simulink library "UsefulBlocksLibrary"  (R2014b)
settings: Solver=ode45  SolverMode=SingleTasking  StartTime=0.0  StopTime=10.0  RelTol=1e-3
undefined symbols (not defined in the file): ActuatorStruct, CalibrationAngles, drivePeakCurrent, JointAbsoluteEncoderCounts_rev, JointPositionGuardMax_rad, JointPositionGuardMin_rad, MotorEncoderCounts_rev, motorTorqueConstant, sampleTime, transmissionRatio
libraries: simulink x13, FM_Library x4, dspsigops x1, simulink_extras x1
(part 1 of 2)
settings Model: Creator=niekbeckers  LastModifiedBy=Administrator
settings OptimizationCC: BlockReduction=off  BooleanDataType=off  UseDivisionForNetSlopeComputation=off  SimCompilerOptimization=off
settings DebuggingCC: SaveWithParameterizedLinksMsg=none  UnderspecifiedInitializationDetection=Classic  MergeDetectMultiDrivingBlocksExec=none  SignalResolutionControl=TryResolveAllWithWarning  SolverPrmCheckMsg=none  FrameProcessingCompatibilityMsg=error  StrictBusMsg=Warning
settings HardwareCC: TargetUnknown=on
settings RTWCC: RTWCompilerOptimization=off
settings ConfigComp: CovMetricSettings=dw  CovHtmlReporting=on  CovSaveCumulativeToWorkspaceVar=on  CovSaveSingleToWorkspaceVar=on  CovModelRefEnable=Off  CovExternalEMLEnable=off  CovSFcnEnable=off

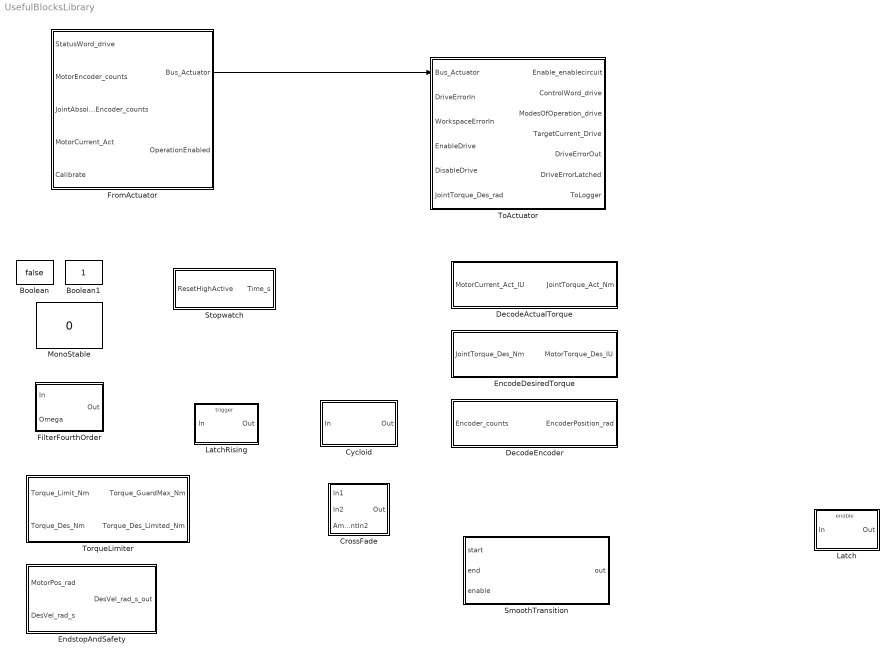
== system UsefulBlocksLibrary ==
  Boolean : Constant  Value=false  OutDataTypeStr=boolean
      settings: OpenFcn=|
      | b = get_param(gcb,'value');
      | if (strcmp(b,'true')),
      |   set_param (gcb,'value','false');
      | else
      |   set_param(gcb,'value','true');
      | end;
  Boolean1 : Constant  OutDataTypeStr=double
      settings: OpenFcn=|
      | b = get_param(gcb,'value');
      | if (strcmp(b,'1')),
      |   set_param (gcb,'value','0');
      | else
      |   set_param(gcb,'value','1');
      | end;
  CrossFade : Subsystem
  Cycloid : Subsystem
  DecodeActualTorque : MATLAB Function  TreatAsAtomicUnit=on  mask(DecodeActualTorque){transmissionRatio=transmissionRatio, motorTorqueConstant=motorTorqueConstant, drivePeakCurrent=drivePeakCurrent}
      mask prompts: transmissionRatio "Transmission ratio (e.g. -8) [-]"; motorTorqueConstant "Motor torque constant [Nm/A]"; drivePeakCurrent "Motor drive peak current Ipeak [A]"
      mask help:
      | Decode Actual Torque value returned from the actuator (motor drive and motor) to torque on the joint (after transmission).
      |
      | Note: due to the way the transmission is set up and the positive motor axis (clockwise is positive as seen from the motor front), there is no need to account for sign change in motor torque or encoder position.
  DecodeEncoder : MATLAB Function  TreatAsAtomicUnit=on  mask(DecodeEncoder){EncoderCounts_rev=MotorEncoderCounts_rev}
      mask prompts: EncoderCounts_rev "Motor encoder increments per revolution (e.g., 8192)"
      mask help: Decode the encoder counts to encoder position in radians
  EncodeDesiredTorque : MATLAB Function  TreatAsAtomicUnit=on  mask(EncodeDesiredTorque){transmissionRatio=transmissionRatio, motorTorqueConstant=motorTorqueConstant, drivePeakCurrent=drivePeakCurrent}
      mask prompts: transmissionRatio "Transmission ratio (e.g. -8) [-]"; motorTorqueConstant "Motor torque constant [Nm/A]"; drivePeakCurrent "Motor drive peak current [A]"
      mask help:
      | Encode desired torque at the joint to torque to be produced by the motor.
      |
      | Note: due to the way the transmission is set up and the positive motor axis (clockwise is positive as seen from the motor front), there is no need to account for sign change in motor torque or encoder position.
  EndstopAndSafety : Subsystem
  FilterFourthOrder : Subsystem
  FromActuator : Subsystem  mask{IdxJoint=1}
      mask prompts: IdxJoint "Actuator joint number (1 = q1, 2 = q5)"
  Latch : Subsystem  mask{ic=0}
      mask prompts: ic "Initial Condition"
  LatchRising : Subsystem  mask{ic=0}
      mask prompts: ic "Initial Condition"
  MonoStable : Constant  Value=0
      settings: OpenFcn=set_param(gcb,'Value','1');tname = ['toggletimer_' gcb];delete(timerfind('name',tname));t = timer('timerfcn', ['set_param(''',gcb,''',''Value'',''0'')'],'executionmode','singleshot','startdelay',1,'name',tname);start(t);
      mask Display: fprintf('PushToTrigger\n%s',get_param(gcb,'value'))
  SmoothTransition : Subsystem
  Stopwatch : Subsystem
  ToActuator : Subsystem  mask{IdxJoint=1}
      mask prompts: IdxJoint "Actuator joint number (1 = q1, 2 = q5)"
  TorqueLimiter : Subsystem
  wires:
  FromActuator/1(Bus_Actuator) -> ToActuator/1(Bus_Actuator)

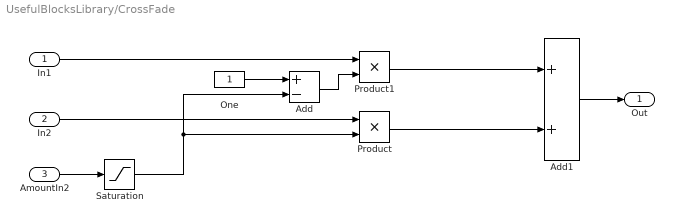
== system UsefulBlocksLibrary/CrossFade ==
  In1 : Inport
  In2 : Inport  Port=2
  AmountIn2 : Inport  Port=3
  Add : Sum  Inputs=+-
  Add1 : Sum
  One : Constant
  Product : Product  RndMeth=Zero
  Product1 : Product  RndMeth=Zero
  Saturation : Saturate  UpperLimit=1  LowerLimit=0
  Out : Outport
  wires:
  In1/1 -> Product1/1
  AmountIn2/1 -> Saturation/1
  One/1 -> Add/1
  Saturation/1 -> Product/2, Add/2
  Add/1 -> Product1/2
  Product/1 -> Add1/2
  Product1/1 -> Add1/1
  In2/1 -> Product/1
  Add1/1 -> Out/1

== system UsefulBlocksLibrary/Cycloid ==
  note: Given a linear input 0<=in<=1, it gives a cycloid output 0<=out<=1.
      | If In is outside the 0..1 range, it is limited to 0 or 1.
  In : Inport
  Gain1 : Gain  Gain=2*pi
  Gain2 : Gain  Gain=1/(2*pi)
  Saturation : Saturate  UpperLimit=1  LowerLimit=0
  Subtract : Sum  Inputs=+-
  Trigonometric Function : Trigonometry
  Out : Outport
  wires:
  Gain1/1 -> Trigonometric Function/1
  Subtract/1 -> Out/1
  In/1 -> Saturation/1
  Saturation/1 -> Gain1/1, Subtract/1
  Trigonometric Function/1 -> Gain2/1
  Gain2/1 -> Subtract/2

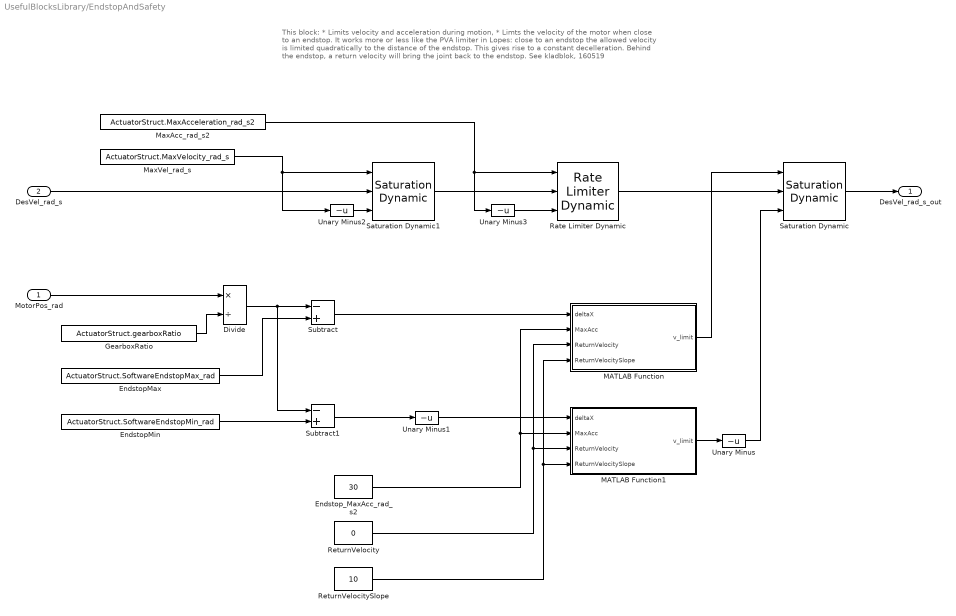
== system UsefulBlocksLibrary/EndstopAndSafety ==
  note: This block:
      | * Limits velocity and acceleration during motion,
      | * Limts the velocity of the motor when close to an endstop. It works more or less like the PVA limiter in Lopes: close to an endstop the allowed velocity is limited quadratically to the distance of the endstop. This gives rise to a constant decelleration. Behind the endstop, a return velocity will bring the joint back to the endstop.  See kladblok, 160519
  MotorPos_rad : Inport
  DesVel_rad_s : Inport  Port=2
  Divide : Product  Inputs=*/
  EndstopMax : Constant  Value=ActuatorStruct.SoftwareEndstopMax_rad
  EndstopMin : Constant  Value=ActuatorStruct.SoftwareEndstopMin_rad
  Endstop_MaxAcc_rad_s2 : Constant  Value=30
  GearboxRatio : Constant  Value=ActuatorStruct.gearboxRatio
  MATLAB Function : MATLAB Function  TreatAsAtomicUnit=on
  MATLAB Function1 : MATLAB Function  TreatAsAtomicUnit=on
  MaxAcc_rad_s2 : Constant  Value=ActuatorStruct.MaxAcceleration_rad_s2
  MaxVel_rad_s : Constant  Value=ActuatorStruct.MaxVelocity_rad_s
  Rate Limiter Dynamic : simulink/Discontinuities/Rate Limiter Dynamic
  ReturnVelocity : Constant  Value=0
  ReturnVelocitySlope : Constant  Value=10
  Saturation Dynamic : simulink/Discontinuities/Saturation Dynamic  OutMin=[]  OutMax=[]  OutDataTypeStr=Inherit: Same as second input  OutDataType=fixdt(1, 16)  OutScaling=2^-10  DoSatur=off
  Saturation Dynamic1 : simulink/Discontinuities/Saturation Dynamic  OutMin=[]  OutMax=[]  OutDataTypeStr=Inherit: Same as second input  OutDataType=fixdt(1, 16)  OutScaling=2^-10  DoSatur=off
  Subtract : Sum  Inputs=-+
  Subtract1 : Sum  Inputs=-+
  Unary Minus{,1..3} (4 alike) : UnaryMinus
  DesVel_rad_s_out : Outport
  wires:
  Unary Minus3/1 -> Rate Limiter Dynamic/3
  MaxAcc_rad_s2/1 -> Rate Limiter Dynamic/1, Unary Minus3/1
  Unary Minus2/1 -> Saturation Dynamic1/3
  MaxVel_rad_s/1 -> Saturation Dynamic1/1, Unary Minus2/1
  DesVel_rad_s/1 -> Saturation Dynamic1/2
  Saturation Dynamic1/1 -> Rate Limiter Dynamic/2
  Rate Limiter Dynamic/1 -> Saturation Dynamic/2
  Saturation Dynamic/1 -> DesVel_rad_s_out/1
  MotorPos_rad/1 -> Divide/1
  GearboxRatio/1 -> Divide/2
  Divide/1 -> Subtract1/1, Subtract/1
  EndstopMax/1 -> Subtract/2
  ReturnVelocitySlope/1 -> MATLAB Function1/4(ReturnVelocitySlope), MATLAB Function/4(ReturnVelocitySlope)
  ReturnVelocity/1 -> MATLAB Function1/3(ReturnVelocity), MATLAB Function/3(ReturnVelocity)
  MATLAB Function/1(v_limit) -> Saturation Dynamic/1
  MATLAB Function1/1(v_limit) -> Unary Minus/1
  Subtract1/1 -> Unary Minus1/1
  EndstopMin/1 -> Subtract1/2
  Endstop_MaxAcc_rad_s2/1 -> MATLAB Function1/2(MaxAcc), MATLAB Function/2(MaxAcc)
  Subtract/1 -> MATLAB Function/1(deltaX)
  Unary Minus/1 -> Saturation Dynamic/3
  Unary Minus1/1 -> MATLAB Function1/1(deltaX)

== system UsefulBlocksLibrary/FilterFourthOrder ==
  In : Inport
  Omega : Inport  Port=2
  Filter1 : MATLAB Function  TreatAsAtomicUnit=on  mask{sampleTime=sampleTime}
      mask prompts: sampleTime "Sample Time"
  Filter2 : MATLAB Function  TreatAsAtomicUnit=on  mask{sampleTime=sampleTime}
      mask prompts: sampleTime "Sample Time"
  Out : Outport
  wires:
  Filter2/1(y) -> Out/1
  In/1 -> Filter1/1(x)
  Omega/1 -> Filter1/2(OmegaFilter), Filter2/2(OmegaFilter)
  Filter1/1(y) -> Filter2/1(x)

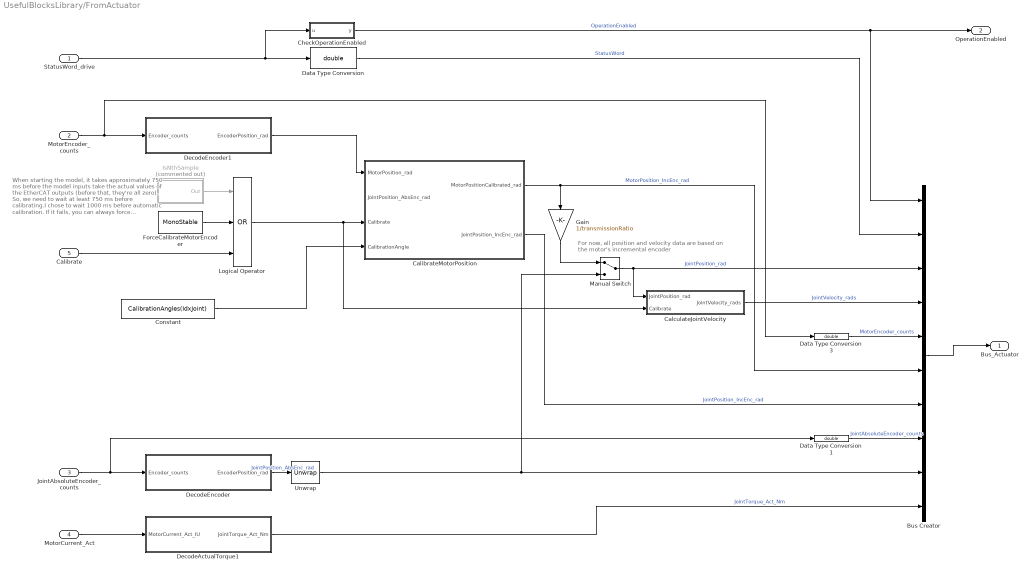
== system UsefulBlocksLibrary/FromActuator ==
  note: For now, all position and velocity data
      | are based on the motor's incremental encoder
  note: When starting the model, it takes approximately 750 ms before the model inputs take the actual values of the EtherCAT outputs (before that, they're all zero). So, we need to wait at least 750 ms before calibrating.I chose to wait 1000 ms before automatic calibration.
      |
      | If it fails, you can always force re-calibration.
  StatusWord_drive : Inport
  MotorEncoder_counts : Inport  Port=2
  JointAbsoluteEncoder_counts : Inport  Port=3
  MotorCurrent_Act : Inport  Port=4
  Calibrate : Inport  Port=5
  Bus Creator : BusCreator  Inputs=10
  CalculateJointVelocity : Subsystem
  "CalibrateMotorPosition    " : MATLAB Function  TreatAsAtomicUnit=on  mask{gearboxRatio=transmissionRatio}
      mask prompts: gearboxRatio "Transmission ratio (e.g. -8) [-]"
  CheckOperationEnabled : MATLAB Function  TreatAsAtomicUnit=on
  Constant : Constant  Value=CalibrationAngles(IdxJoint)
  Data Type Conversion : DataTypeConversion  OutDataTypeStr=double
  Data Type Conversion1 : DataTypeConversion  OutDataTypeStr=double
  Data Type Conversion3 : DataTypeConversion  OutDataTypeStr=double
  DecodeActualTorque1 : MATLAB Function  TreatAsAtomicUnit=on  mask(DecodeActualTorque){transmissionRatio=transmissionRatio, motorTorqueConstant=motorTorqueConstant, drivePeakCurrent=drivePeakCurrent}
      mask prompts: transmissionRatio "Transmission ratio (e.g. -8) [-]"; motorTorqueConstant "Motor torque constant [Nm/A]"; drivePeakCurrent "Motor drive peak current Ipeak [A]"
      mask help:
      | Decode Actual Torque value returned from the actuator (motor drive and motor) to torque on the joint (after transmission).
      |
      | Note: due to the way the transmission is set up and the positive motor axis (clockwise is positive as seen from the motor front), there is no need to account for sign change in motor torque or encoder position.
  DecodeEncoder : MATLAB Function  TreatAsAtomicUnit=on  mask(DecodeEncoder){EncoderCounts_rev=JointAbsoluteEncoderCounts_rev}
      mask prompts: EncoderCounts_rev "Motor encoder increments per revolution (e.g., 8192)"
      mask help: Decode the encoder counts to encoder position in radians
  DecodeEncoder1 : MATLAB Function  TreatAsAtomicUnit=on  mask(DecodeEncoder){EncoderCounts_rev=MotorEncoderCounts_rev}
      mask prompts: EncoderCounts_rev "Motor encoder increments per revolution (e.g., 8192)"
      mask help: Decode the encoder counts to encoder position in radians
  ForceCalibrateMotorEncoder : FM_Library/MonoStable  Value=0  OutMin=[]  OutMax=[]  OutDataTypeStr=Inherit: Inherit from 'Constant value'
  Gain : Gain  Gain=1/transmissionRatio
  IsNthSample : Subsystem  Commented=on  InitFcn=|  mask{N=1000}
      | return; %Disable this becasue it doesnt work!                                                                                                                                                          
      | h = gcb;                                                                                                                                                                                               
      | n = 0; % Number of enable blocks detected upstream                                                                                                                                                     
      | t = []; % type of enable blocks                                                                                                                                                                        
      | while 1,                                                                                                                                                                                               
      |   % Find parent                                                                                                                                                                                        
      |   h = get_param(h,'parent');                                                                                                                                                                           
      |   if (strcmp(h,'')),                                                                                                                                                                                   
      |       % Then we've reached the root                                                                                                                                                                    
      |       break;                                                                                                                                                                                           
      |   end;                                                                                                                                                                                                 
      |   % and check if it has an enable port                                                                                                                                                                 
      |   e = find_system(h,'searchdepth',1, 'BlockType','EnablePort');                                                                                                                                        
      |   if (numel(e)==1),                                                                                                                                                                                    
      |     s = get_param(e{1},'StatesWhenEnabling');                                                                                                                                                          
      |     n=n+1;                                                                                                                                                                                             
      |     if (strcmp(s,'held')),                                                                                                                                                                             
      |         t=[t;'h']; %#ok<AGROW>                                                                                                                                                                         
      |     else                                                                                                                                                                                               
      |         t=[t;'r']; %#ok<AGROW>                                                                                                                                                                         
      |     end;                                                                                                                                                                                               
      |   elseif (numel(e)>1),                                                                                                                                                                                 
      |       error('hun? Multiple enable blocks!')                                                                                                                                                            
      |   end;                                                                                                                                                                                                 
      | end;                                                                                                                                                                                                   
      |                                                                                                                                                                                                        
      | if (n==0),                                                                                                                                                                                             
      |     warning('Warning: %s - The block is not inside an enabled block',gcb)                                                                                                                              
      | elseif (n==1),                                                                                                                                                                                         
      |     if (t(1)=='r')                                                                                                                                                                                     
      |         % This is okay, do nothing                                                                                                                                                                     
      |     else                                                                                                                                                                                               
      |         warning('Warning: %s - This block is inside an enabled block which has its "State when enabling" set to "held". Usually you want it set to "reset" for correct operation.',gcb);               
      |     end;                                                                                                                                                                                               
      | else % n>1                                                                                                                                                                                             
      |     warning('Warning: %s - This block is inside multiple nested enabled blocks. Check which blocks are "held" and which are "reset". You usually want to have at least one "reset" enabled block',gcb);
      | end;
  Logical Operator : Logic  Operator=OR  Inputs=3  AllPortsSameDT=off  OutDataTypeStr=boolean
  Manual Switch : ManualSwitch
  Unwrap : dspsigops/Unwrap  tol=pi  InputProcessing=Columns as channels (frame based)  running=off
  Bus_Actuator : Outport
  OperationEnabled : Outport  Port=2
  wires:
  Logical Operator/1 -> CalculateJointVelocity/2(Calibrate), "CalibrateMotorPosition    "/3(Calibrate)
  Bus Creator/1 -> Bus_Actuator/1
  Data Type Conversion3/1 -> Bus Creator/5  "MotorEncoder_counts"
  MotorEncoder_counts/1 -> DecodeEncoder1/1(Encoder_counts), Data Type Conversion3/1
  Manual Switch/1 -> CalculateJointVelocity/1(JointPosition_rad), Bus Creator/3  "JointPosition_rad"
  Data Type Conversion/1 -> Bus Creator/2  "StatusWord"
  ForceCalibrateMotorEncoder/1 -> Logical Operator/2
  Data Type Conversion1/1 -> Bus Creator/8  "JointAbsoluteEncoder_counts"
  "CalibrateMotorPosition    "/2(JointPosition_IncEnc_rad) -> Bus Creator/7  "JointPosition_IncEnc_rad"
  JointAbsoluteEncoder_counts/1 -> DecodeEncoder/1(Encoder_counts), Data Type Conversion1/1
  IsNthSample/1(Out) -> Logical Operator/1
  CheckOperationEnabled/1(y) -> OperationEnabled/1, Bus Creator/1  "OperationEnabled"
  MotorCurrent_Act/1 -> DecodeActualTorque1/1(MotorCurrent_Act_IU)
  DecodeEncoder1/1(EncoderPosition_rad) -> "CalibrateMotorPosition    "/1(MotorPosition_rad)
  StatusWord_drive/1 -> CheckOperationEnabled/1(u), Data Type Conversion/1
  DecodeActualTorque1/1(JointTorque_Act_Nm) -> Bus Creator/10  "JointTorque_Act_Nm"
  "CalibrateMotorPosition    "/1(MotorPositionCalibrated_rad) -> Gain/1, Bus Creator/6  "MotorPosition_IncEnc_rad"
  DecodeEncoder/1(EncoderPosition_rad) -> Unwrap/1  "JointPosition_AbsEnc_rad"
  CalculateJointVelocity/1(JointVelocity_rads) -> Bus Creator/4  "JointVelocity_rads"
  Constant/1 -> "CalibrateMotorPosition    "/4(CalibrationAngle)
  Calibrate/1 -> Logical Operator/3
  Gain/1 -> Manual Switch/1
  Unwrap/1 -> Manual Switch/2, Bus Creator/9

== system UsefulBlocksLibrary/Latch ==
  note: Enable == HIGH: OUtput follows input
      | Enable == LOW: Output does not change anymore.
  In : Inport
  Enable : EnablePort
  Out : Outport  InitialOutput=ic
  wires:
  In/1 -> Out/1

== system UsefulBlocksLibrary/LatchRising ==
  note: Enable == HIGH: OUtput follows input
      | Enable == LOW: Output does not change anymore.
  In : Inport
  Trigger : TriggerPort  PortDimensions=1
  Out : Outport  InitialOutput=ic
  wires:
  In/1 -> Out/1

== system UsefulBlocksLibrary/SmoothTransition ==
  start : Inport
  end : Inport  Port=2
  enable : Inport  Port=3
  Add : Sum
  Subsystem : Subsystem  mask{Ts=0.001, Ttransition=5}
      mask prompts: Ts "Sample time [s]"; Ttransition "Transition time"
  out : Outport  SourceOfInitialOutputValue=Input signal
  wires:
  end/1 -> Subsystem/2(end)
  enable/1 -> Subsystem/Enable
  Subsystem/1("out ") -> Add/2
  Add/1 -> out/1
  start/1 -> Subsystem/1(start), Add/1

== system UsefulBlocksLibrary/Stopwatch ==
  note: Stopwatch -
      | Outputs time in seconds.
      | Reset during high level of Rest pulse
  ResetHighActive : Inport
  Counter Free-Running : simulink/Sources/Counter Free-Running  NumBits=32  tsamp=-1
  Data Type Conversion : DataTypeConversion  OutDataTypeStr=double
  LatchRising : FM_Library/LatchRising  ic=0
  Subtract : Sum  Inputs=-+
  sample time : Gain  Gain=sampleTime
  Time_s : Outport
  wires:
  ResetHighActive/1 -> LatchRising/Trigger
  Data Type Conversion/1 -> sample time/1
  sample time/1 -> Time_s/1
  Subtract/1 -> Data Type Conversion/1
  Counter Free-Running/1 -> LatchRising/1, Subtract/2
  LatchRising/1 -> Subtract/1  "startTime"

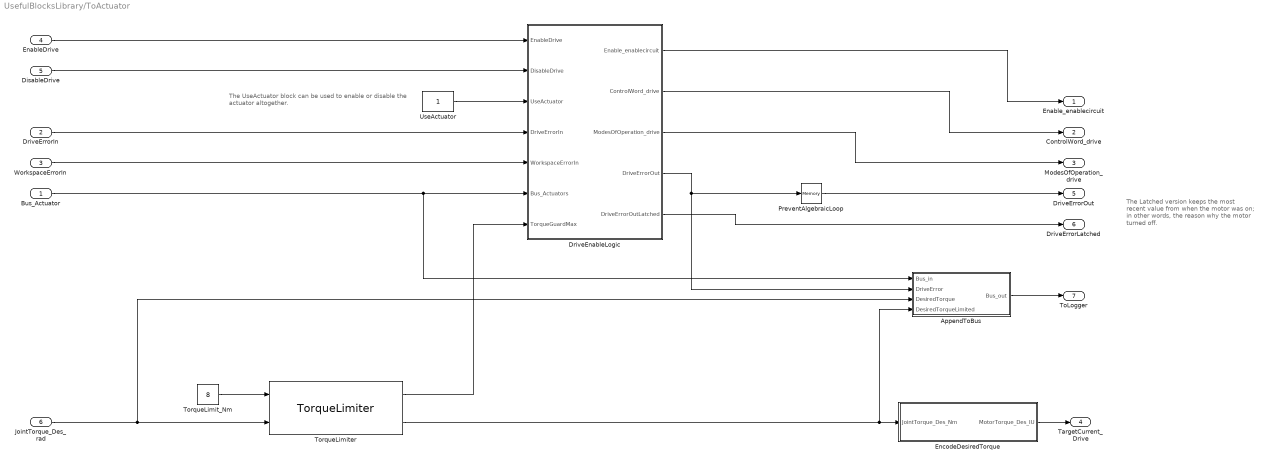
== system UsefulBlocksLibrary/ToActuator ==
  note: The UseActuator block can be used to enable or disable the actuator altogether.
  note: The Latched version keeps the most recent value from when the motor was on; in other words, the reason why the motor turned off.
  Bus_Actuator : Inport
  DriveErrorIn : Inport  Port=2
  WorkspaceErrorIn : Inport  Port=3
  EnableDrive : Inport  Port=4
  DisableDrive : Inport  Port=5
  JointTorque_Des_rad : Inport  Port=6
  AppendToBus : Subsystem
  DriveEnableLogic : Subsystem
  EncodeDesiredTorque : MATLAB Function  TreatAsAtomicUnit=on  mask(EncodeDesiredTorque){transmissionRatio=transmissionRatio, motorTorqueConstant=motorTorqueConstant, drivePeakCurrent=drivePeakCurrent}
      mask prompts: transmissionRatio "Transmission ratio (e.g. -8) [-]"; motorTorqueConstant "Motor torque constant [Nm/A]"; drivePeakCurrent "Motor drive peak current [A]"
      mask help:
      | Encode desired torque at the joint to torque to be produced by the motor.
      |
      | Note: due to the way the transmission is set up and the positive motor axis (clockwise is positive as seen from the motor front), there is no need to account for sign change in motor torque or encoder position.
  PreventAlgebraicLoop : Memory
  TorqueLimit_Nm : Constant  Value=8
  TorqueLimiter : FM_Library/TorqueLimiter
  UseActuator : Constant  OutDataTypeStr=double
      settings: OpenFcn=|
      | b = get_param(gcb,'value');
      | if (strcmp(b,'1')),
      |   set_param (gcb,'value','0');
      | else
      |   set_param(gcb,'value','1');
      | end;
  Enable_enablecircuit : Outport
  ControlWord_drive : Outport  Port=2
  ModesOfOperation_drive : Outport  Port=3
  TargetCurrent_Drive : Outport  Port=4
  DriveErrorOut : Outport  Port=5
  DriveErrorLatched : Outport  Port=6
  ToLogger : Outport  Port=7
  wires:
  UseActuator/1 -> DriveEnableLogic/3(UseActuator)
  AppendToBus/1(Bus_out) -> ToLogger/1
  PreventAlgebraicLoop/1 -> DriveErrorOut/1
  DriveErrorIn/1 -> DriveEnableLogic/4(DriveErrorIn)
  DriveEnableLogic/4(DriveErrorOut) -> PreventAlgebraicLoop/1, AppendToBus/2(DriveError)
  DisableDrive/1 -> DriveEnableLogic/2(DisableDrive)
  EnableDrive/1 -> DriveEnableLogic/1(EnableDrive)
  Bus_Actuator/1 -> AppendToBus/1(Bus_in), DriveEnableLogic/6(Bus_Actuators)
  EncodeDesiredTorque/1(MotorTorque_Des_IU) -> TargetCurrent_Drive/1
  DriveEnableLogic/2(ControlWord_drive) -> ControlWord_drive/1
  DriveEnableLogic/3(ModesOfOperation_drive) -> ModesOfOperation_drive/1
  TorqueLimit_Nm/1 -> TorqueLimiter/1
  DriveEnableLogic/5(DriveErrorOutLatched) -> DriveErrorLatched/1
  TorqueLimiter/2 -> EncodeDesiredTorque/1(JointTorque_Des_Nm), AppendToBus/4(DesiredTorqueLimited)
  TorqueLimiter/1 -> DriveEnableLogic/7(TorqueGuardMax)
  JointTorque_Des_rad/1 -> TorqueLimiter/2, AppendToBus/3(DesiredTorque)
  DriveEnableLogic/1(Enable_enablecircuit) -> Enable_enablecircuit/1
  WorkspaceErrorIn/1 -> DriveEnableLogic/5(WorkspaceErrorIn)

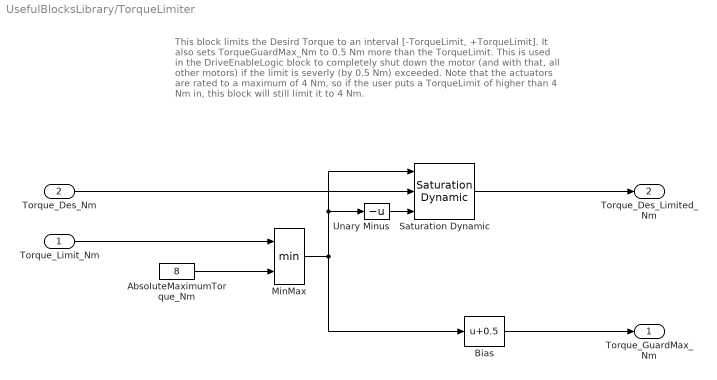
== system UsefulBlocksLibrary/TorqueLimiter ==
  note: This block limits the Desird Torque to an interval [-TorqueLimit, +TorqueLimit]. It also sets TorqueGuardMax_Nm to 0.5 Nm more than the TorqueLimit. This is used in the DriveEnableLogic block to completely shut down the motor (and with that, all other motors) if the limit is severly (by 0.5 Nm) exceeded.
      |
      | Note that the actuators are rated to a maximum of 4 Nm, so if the user puts a TorqueLimit of higher than 4 Nm in, this block will still limit it to 4 Nm.
  Torque_Limit_Nm : Inport
  Torque_Des_Nm : Inport  Port=2
  AbsoluteMaximumTorque_Nm : Constant  Value=8
  Bias : Bias  Bias=0.5
  MinMax : MinMax  Inputs=2
  Saturation Dynamic : simulink/Discontinuities/Saturation Dynamic  OutMin=[]  OutMax=[]  OutDataTypeStr=Inherit: Same as second input  OutDataType=fixdt(1, 16)  OutScaling=2^-10  DoSatur=off
  Unary Minus : UnaryMinus
  Torque_GuardMax_Nm : Outport
  Torque_Des_Limited_Nm : Outport  Port=2
  wires:
  Torque_Limit_Nm/1 -> MinMax/1
  AbsoluteMaximumTorque_Nm/1 -> MinMax/2
  MinMax/1 -> Bias/1, Unary Minus/1, Saturation Dynamic/1
  Unary Minus/1 -> Saturation Dynamic/3
  Saturation Dynamic/1 -> Torque_Des_Limited_Nm/1
  Torque_Des_Nm/1 -> Saturation Dynamic/2
  Bias/1 -> Torque_GuardMax_Nm/1

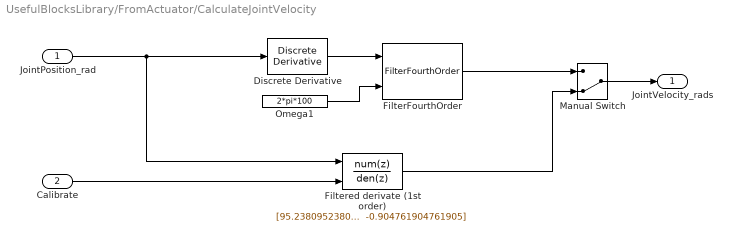
== system UsefulBlocksLibrary/FromActuator/CalculateJointVelocity ==
  JointPosition_rad : Inport
  Calibrate : Inport  Port=2
  Discrete Derivative : simulink/Discrete/Discrete Derivative  gainval=1.0  ICPrevScaledInput=0.0  InputProcessing=Inherited  OutMin=[]  OutMax=[]  OutDataType=fixdt(1, 16)  OutScaling=2^-10  DoSatur=off
  FilterFourthOrder : FM_Library/FilterFourthOrder
  Filtered derivate (1st order) : DiscreteTransferFcn  Numerator=[95.238095238095241 -95.238095238095241]  Denominator="[1.000000000000000  -0.904761904761905]"  ExternalReset=Rising
      settings: InputPortMap=u0,r7
  Manual Switch : ManualSwitch  CurrentSetting=0
  Omega1 : Constant  Value=2*pi*100  OutDataTypeStr=double
  JointVelocity_rads : Outport
  wires:
  Omega1/1 -> FilterFourthOrder/2
  Discrete Derivative/1 -> FilterFourthOrder/1
  FilterFourthOrder/1 -> Manual Switch/1
  Manual Switch/1 -> JointVelocity_rads/1
  Calibrate/1 -> Filtered derivate (1st order)/2
  Filtered derivate (1st order)/1 -> Manual Switch/2
  JointPosition_rad/1 -> Filtered derivate (1st order)/1, Discrete Derivative/1

== system UsefulBlocksLibrary/FromActuator/IsNthSample ==
  note: This block outputs 1 on the Nth sample of the enabled block,
      | zero otherwise. Note that this is 0-based (e.g., N=3 is the fourth
      | sample). Note that it only works if the enable port has
      | "States when enabled" set to "reset"!
  Counter Free-Running : simulink/Sources/Counter Free-Running  NumBits=16  tsamp=-1
  N : Constant  Value=N
  Relational Operator : RelationalOperator  Operator===  OutDataTypeStr=boolean
  Out : Outport
  wires:
  N/1 -> Relational Operator/2
  Counter Free-Running/1 -> Relational Operator/1
  Relational Operator/1 -> Out/1

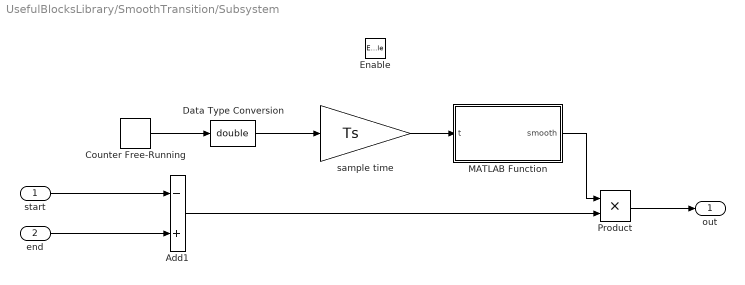
== system UsefulBlocksLibrary/SmoothTransition/Subsystem ==
  start : Inport
  end : Inport  Port=2
  Enable : EnablePort
  Add1 : Sum  Inputs=-+
  Counter Free-Running : simulink/Sources/Counter Free-Running  NumBits=16  tsamp=-1
  Data Type Conversion : DataTypeConversion  OutDataTypeStr=double
  MATLAB Function : MATLAB Function  TreatAsAtomicUnit=on
  Product : Product
  sample time : Gain  Gain=Ts
  "out " : Outport
  wires:
  sample time/1 -> MATLAB Function/1(t)
  MATLAB Function/1(smooth) -> Product/1
  Add1/1 -> Product/2
  Product/1 -> "out "/1
  start/1 -> Add1/1
  Data Type Conversion/1 -> sample time/1
  Counter Free-Running/1 -> Data Type Conversion/1
  end/1 -> Add1/2

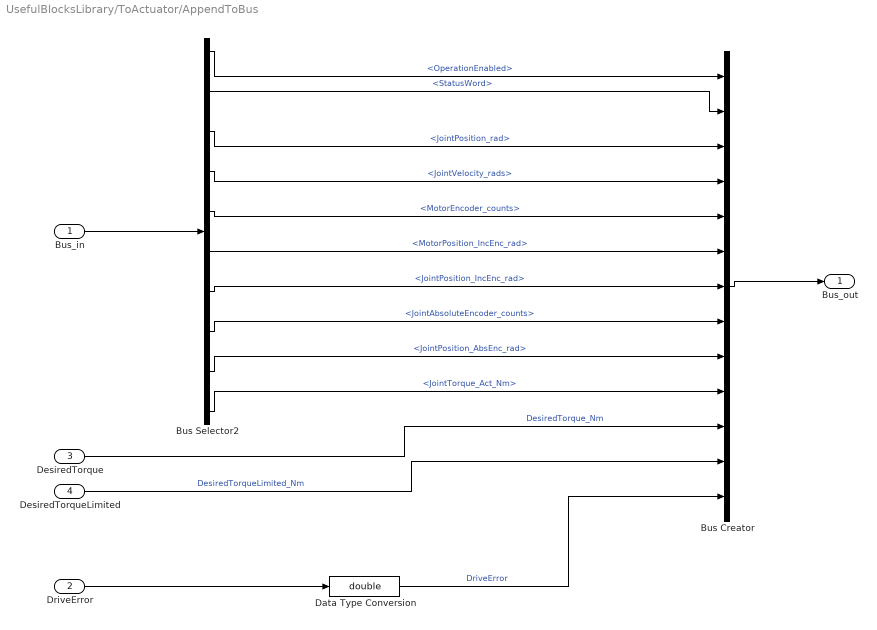
== system UsefulBlocksLibrary/ToActuator/AppendToBus ==
  Bus_in : Inport
  DriveError : Inport  Port=2
  DesiredTorque : Inport  Port=3
  DesiredTorqueLimited : Inport  Port=4
  Bus Creator : BusCreator  Inputs=13
  Bus Selector2 : BusSelector  OutputSignals=OperationEnabled,StatusWord,JointPosition_rad,JointVelocity_rads,MotorEncoder_counts,MotorPosition_IncEnc_rad,JointPosition_IncEnc_rad,JointAbsoluteEncoder_counts,JointPosition_AbsEnc_rad,JointTorque_Act_Nm
  Data Type Conversion : DataTypeConversion  OutDataTypeStr=double
  Bus_out : Outport
  wires:
  Bus Selector2/6 -> Bus Creator/6  "<MotorPosition_IncEnc_rad>"
  Bus Selector2/9 -> Bus Creator/9  "<JointPosition_AbsEnc_rad>"
  Bus Selector2/8 -> Bus Creator/8  "<JointAbsoluteEncoder_counts>"
  Bus Selector2/7 -> Bus Creator/7  "<JointPosition_IncEnc_rad>"
  Bus Selector2/5 -> Bus Creator/5  "<MotorEncoder_counts>"
  Bus Selector2/4 -> Bus Creator/4  "<JointVelocity_rads>"
  Bus Selector2/3 -> Bus Creator/3  "<JointPosition_rad>"
  Bus Selector2/2 -> Bus Creator/2  "<StatusWord>"
  Bus Selector2/1 -> Bus Creator/1  "<OperationEnabled>"
  DesiredTorqueLimited/1 -> Bus Creator/12  "DesiredTorqueLimited_Nm"
  DesiredTorque/1 -> Bus Creator/11  "DesiredTorque_Nm"
  Data Type Conversion/1 -> Bus Creator/13  "DriveError"
  DriveError/1 -> Data Type Conversion/1
  Bus_in/1 -> Bus Selector2/1
  Bus Creator/1 -> Bus_out/1
  Bus Selector2/10 -> Bus Creator/10  "<JointTorque_Act_Nm>"

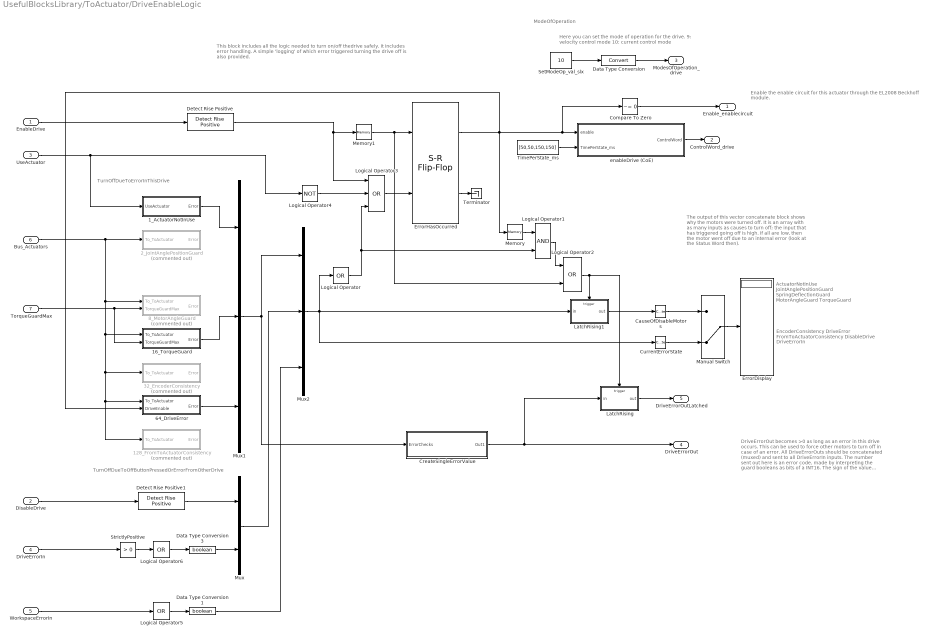
== system UsefulBlocksLibrary/ToActuator/DriveEnableLogic ==
  note: Enable the enable circuit for this actuator through the EL2008
      | Beckhoff module.
  note: ModeOfOperation
  note: ActuatorNotInUse
      | JointAnglePositionGuard
      | SpringDeflectionGuard
      | MotorAngleGuard
      | TorqueGuard
  note: EncoderConsistency
      | DriveError
      | FromToActuatorConsistency
      | DisableDrive
      | DriveErrorIn
  note: DriveErrorOut becomes >0 as long as an error in this drive occurs. This can be used to force other motors to turn off in case of an error.
      | All DriveErrorOuts should be concatenated (muxed)  and sent to all DriveErrorIn inputs. The number sent out here is an error code, made by interpreting the guard booleans as bits of a INT16.
      | The sign of the value indicates:
      | >=0: UseActuator=true
      | <0: UseActuator = False
  note: TurnOffDueToOffButtonPressedOrErrorFromOtherDrive
  note: TurnOffDueToErrorInThisDrive
  note: This block includes all the logic needed to turn on/off thedrive safely. It includes error handling. A simple 'logging' of which error triggered turning the drive off is also provided.
  note: The output of this vector concatenate block shows why the motors were turned off. It is an array with as many inputs as causes to turn off; the input that has triggered going off is high. If all are low, then the motor went off due to an internal error (look at the Status Word then).
  note: Here you can set the mode of operation for the drive.
      | 9: velocity control mode
      | 10: current control mode
  EnableDrive : Inport
  DisableDrive : Inport  Port=2
  UseActuator : Inport  Port=3
  DriveErrorIn : Inport  Port=4
  WorkspaceErrorIn : Inport  Port=5
  Bus_Actuators : Inport  Port=6
  TorqueGuardMax : Inport  Port=7
  128_FromToActuatorConsistency : Subsystem  Commented=on
  16_TorqueGuard : Subsystem
  1_ActuatorNotInUse : Subsystem
  2_JointAnglePositionGuard : Subsystem  Commented=on
  32_EncoderConsistency : Subsystem  Commented=on
  64_DriveError : Subsystem
  8_MotorAngleGuard : Subsystem  Commented=on
  CauseOfDisableMotors : Concatenate  NumInputs=1
  Compare To Zero : simulink/Logic and Bit Operations/Compare To Zero  relop=~=  OutDataTypeStr=boolean
  CreateSingleErrorValue : Subsystem
  CurrentErrorState : Concatenate  NumInputs=1
  Data Type Conversion : DataTypeConversion
  Data Type Conversion1 : DataTypeConversion  OutDataTypeStr=boolean
  Data Type Conversion3 : DataTypeConversion  OutDataTypeStr=boolean
  Detect Rise Positive : simulink/Logic and Bit Operations/Detect Rise Positive  vinit=0  InputProcessing=Inherited  OutDataTypeStr=boolean
  Detect Rise Positive1 : simulink/Logic and Bit Operations/Detect Rise Positive  vinit=0  InputProcessing=Inherited  OutDataTypeStr=boolean
  ErrorDisplay : Display
  ErrorHasOccurred : simulink_extras/Flip Flops/S-R Flip-Flop  initial_condition=0
  LatchRising : Subsystem  TreatAsAtomicUnit=on
  LatchRising1 : Subsystem  TreatAsAtomicUnit=on
  Logical Operator : Logic  Operator=OR  Inputs=1  AllPortsSameDT=off  OutDataTypeStr=boolean
  Logical Operator1 : Logic  AllPortsSameDT=off  OutDataTypeStr=boolean
  Logical Operator2 : Logic  Operator=OR  AllPortsSameDT=off  OutDataTypeStr=boolean
  Logical Operator3 : Logic  Operator=OR  Inputs=3  AllPortsSameDT=off  OutDataTypeStr=boolean
  Logical Operator4 : Logic  Operator=NOT  Inputs=1  AllPortsSameDT=off  OutDataTypeStr=boolean
  Logical Operator5 : Logic  Operator=OR  Inputs=1  AllPortsSameDT=off  OutDataTypeStr=boolean
  Logical Operator6 : Logic  Operator=OR  Inputs=1  AllPortsSameDT=off  OutDataTypeStr=boolean
  Manual Switch : ManualSwitch  CurrentSetting=0
  Memory : Memory
  Memory1 : Memory
  Mux : Mux  Inputs=2
  Mux1 : Mux  Inputs=3
  Mux2 : Mux  Inputs=3
  SetModeOp_val_slx : Constant  Value=10
  StrictlyPositive : simulink/Logic and Bit Operations/Compare To Zero  relop=>  OutDataTypeStr=boolean
  Terminator : Terminator
  TimePerState_ms : Constant  Value=[50,50,150,150]
  enableDrive (CoE) : MATLAB Function  TreatAsAtomicUnit=on
  Enable_enablecircuit : Outport
  ControlWord_drive : Outport  Port=2
  ModesOfOperation_drive : Outport  Port=3
  DriveErrorOut : Outport  Port=4
  DriveErrorOutLatched : Outport  Port=5
  wires:
  LatchRising/1(out) -> DriveErrorOutLatched/1
  CreateSingleErrorValue/1(Out1) -> DriveErrorOut/1, LatchRising/1(in)
  StrictlyPositive/1 -> Logical Operator6/1
  TorqueGuardMax/1 -> 16_TorqueGuard/2(TorqueGuardMax), 8_MotorAngleGuard/2(TorqueGuardMax)
  LatchRising1/1(out) -> CauseOfDisableMotors/1
  Logical Operator/1 -> Logical Operator3/3, Logical Operator1/2
  SetModeOp_val_slx/1 -> Data Type Conversion/1
  EnableDrive/1 -> Detect Rise Positive/1
  enableDrive (CoE)/1(ControlWord) -> ControlWord_drive/1
  ErrorHasOccurred/1 -> Memory/1, 64_DriveError/2(DriveEnable), Compare To Zero/1, enableDrive (CoE)/1(enable)
  Mux2/1 -> Logical Operator/1, CurrentErrorState/1, LatchRising1/1(in)
  Detect Rise Positive1/1 -> Mux/1
  DisableDrive/1 -> Detect Rise Positive1/1
  ErrorHasOccurred/2 -> Terminator/1
  Data Type Conversion/1 -> ModesOfOperation_drive/1
  CauseOfDisableMotors/1 -> Manual Switch/1
  Memory1/1 -> Logical Operator2/2, ErrorHasOccurred/1
  Memory/1 -> Logical Operator1/1
  Logical Operator2/1 -> LatchRising1/Trigger, LatchRising/Trigger
  CurrentErrorState/1 -> Manual Switch/2
  Logical Operator1/1 -> Logical Operator2/1
  Manual Switch/1 -> ErrorDisplay/1
  Logical Operator3/1 -> ErrorHasOccurred/2
  Detect Rise Positive/1 -> Logical Operator3/1, Memory1/1
  TimePerState_ms/1 -> enableDrive (CoE)/2(TimePerState_ms)
  UseActuator/1 -> 1_ActuatorNotInUse/1(UseActuator), Logical Operator4/1
  DriveErrorIn/1 -> StrictlyPositive/1
  Logical Operator6/1 -> Data Type Conversion3/1
  Mux/1 -> Mux2/2
  Bus_Actuators/1 -> 2_JointAnglePositionGuard/1(To_ToActuator), 8_MotorAngleGuard/1(To_ToActuator), 16_TorqueGuard/1(To_ToActuator), 128_FromToActuatorConsistency/1(To_ToActuator), 64_DriveError/1(To_ToActuator), 32_EncoderConsistency/1(To_ToActuator)
  Logical Operator4/1 -> Logical Operator3/2
  1_ActuatorNotInUse/1(Error) -> Mux1/1
  64_DriveError/1(Error) -> Mux1/3
  16_TorqueGuard/1(Error) -> Mux1/2
  Compare To Zero/1 -> Enable_enablecircuit/1
  Data Type Conversion3/1 -> Mux/2
  Logical Operator5/1 -> Data Type Conversion1/1
  WorkspaceErrorIn/1 -> Logical Operator5/1
  Mux1/1 -> CreateSingleErrorValue/1(ErrorChecks), Mux2/1
  Data Type Conversion1/1 -> Mux2/3

== system UsefulBlocksLibrary/ToActuator/DriveEnableLogic/128_FromToActuatorConsistency ==
  note: This block checks whether the FromActuator and ToActuator blocks use the same ActuatorStruct. If not, you've done something wrong. It does this by checking if the JointEncoderOffsets are identical.
  To_ToActuator : Inport
  Bus Selector : BusSelector  OutputSignals=JointEncoderOffset
  Constant : Constant  Value=ActuatorStruct.JointEncoderOffset
  Relational Operator : RelationalOperator  Operator=~=  OutDataTypeStr=boolean
  Error : Outport
  wires:
  To_ToActuator/1 -> Bus Selector/1
  Relational Operator/1 -> Error/1
  Bus Selector/1 -> Relational Operator/1  "<JointEncoderOffset>"
  Constant/1 -> Relational Operator/2

== system UsefulBlocksLibrary/ToActuator/DriveEnableLogic/16_TorqueGuard ==
  To_ToActuator : Inport
  TorqueGuardMax : Inport  Port=2
  Abs : Abs
  Bus Selector : BusSelector  OutputSignals=JointTorque_Act_Nm
  Relational Operator : RelationalOperator  Operator=>  OutDataTypeStr=boolean
  Error : Outport  PortDimensions=1
  wires:
  TorqueGuardMax/1 -> Relational Operator/2
  Bus Selector/1 -> Abs/1  "<JointTorque_Act_Nm>"
  To_ToActuator/1 -> Bus Selector/1
  Abs/1 -> Relational Operator/1
  Relational Operator/1 -> Error/1

== system UsefulBlocksLibrary/ToActuator/DriveEnableLogic/1_ActuatorNotInUse ==
  note: When UseActuator = 0, this block outputs 1. Later in the chain, the ErrorValue is then negated, resulting in -1 if there are no other errors. Note, thus, that this output does not really indicate an error; more a status.
  UseActuator : Inport
  Logical Operator1 : Logic  Operator=NOT  AllPortsSameDT=off  OutDataTypeStr=boolean
  Error : Outport  PortDimensions=1
  wires:
  Logical Operator1/1 -> Error/1
  UseActuator/1 -> Logical Operator1/1

== system UsefulBlocksLibrary/ToActuator/DriveEnableLogic/2_JointAnglePositionGuard ==
  note: This block makes sure that the motors are turned off (and cannot go on) when the joint is outside its normal range.
  To_ToActuator : Inport
  Bus Selector : BusSelector  OutputSignals=JointPosition_rad
  Logical Operator : Logic  Operator=OR  AllPortsSameDT=off  OutDataTypeStr=boolean
  Maximum : Constant  Value=JointPositionGuardMax_rad(IdxJoint)
  Minimum : Constant  Value=JointPositionGuardMin_rad(IdxJoint)
  Relational Operator : RelationalOperator  Operator=<=  OutDataTypeStr=boolean
  Relational Operator1 : RelationalOperator  OutDataTypeStr=boolean
  Error : Outport
  wires:
  To_ToActuator/1 -> Bus Selector/1
  Relational Operator/1 -> Logical Operator/1
  Relational Operator1/1 -> Logical Operator/2
  Logical Operator/1 -> Error/1
  Minimum/1 -> Relational Operator/2
  Maximum/1 -> Relational Operator1/2
  Bus Selector/1 -> Relational Operator1/1, Relational Operator/1  "<JointPosition_rad>"

== system UsefulBlocksLibrary/ToActuator/DriveEnableLogic/32_EncoderConsistency ==
  note: This block checks whether the three encoders are consistent. Ideally, the sum (with jointAngle negated) should be exactly zero at all times (also when forces are exerted). We allow some room around it however.
  To_ToActuator : Inport
  Abs : Abs
  Add : Sum  Inputs=+-
  Bus Selector : BusSelector  OutputSignals=JointPosition_IncEnc_rad,JointPosition_AbsEnc_rad
  Compare To Constant : simulink/Logic and Bit Operations/Compare To Constant  relop=<=  const=3.0  OutDataTypeStr=boolean
  EncoderInConsistency_rad : Concatenate  NumInputs=1
  Error : Outport
  wires:
  Bus Selector/1 -> Add/1  "<JointPosition_IncEnc_rad>"
  To_ToActuator/1 -> Bus Selector/1
  Compare To Constant/1 -> Error/1
  Abs/1 -> Compare To Constant/1
  Bus Selector/2 -> Add/2  "<JointPosition_AbsEnc_rad>"
  Add/1 -> EncoderInConsistency_rad/1
  EncoderInConsistency_rad/1 -> Abs/1

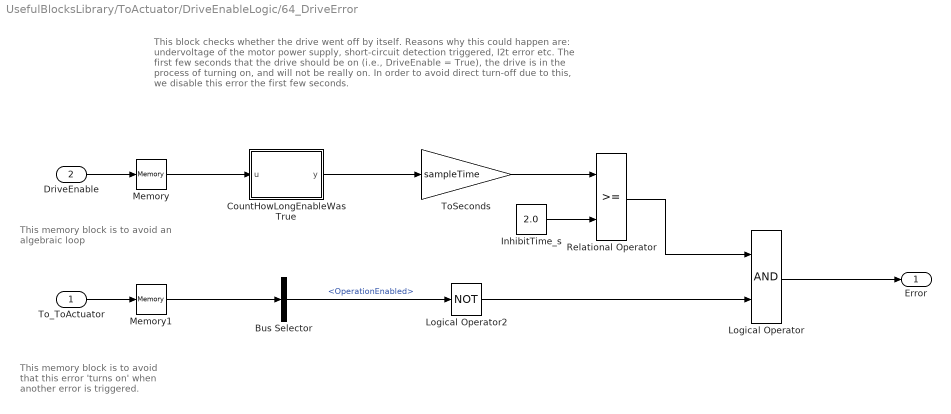
== system UsefulBlocksLibrary/ToActuator/DriveEnableLogic/64_DriveError ==
  note: This memory block is to avoid that this error 'turns on' when another error is triggered.
  note: This memory block is to avoid an
      | algebraic loop
  note: This block checks whether the drive went off by itself. Reasons why this could happen are: undervoltage of the motor power supply, short-circuit detection triggered, I2t error etc.
      | The first few seconds that the drive should be on (i.e., DriveEnable = True), the drive is in the process of turning on, and will not be really on. In order to avoid direct turn-off due to this, we disable this error the first few seconds.
  To_ToActuator : Inport
  DriveEnable : Inport  Port=2
  Bus Selector : BusSelector  OutputSignals=OperationEnabled
  CountHowLongEnableWasTrue : MATLAB Function  TreatAsAtomicUnit=on
  InhibitTime_s : Constant  Value=2.0
  Logical Operator : Logic  AllPortsSameDT=off  OutDataTypeStr=boolean
  Logical Operator2 : Logic  Operator=NOT  AllPortsSameDT=off  OutDataTypeStr=boolean
  Memory : Memory
  Memory1 : Memory
  Relational Operator : RelationalOperator  OutDataTypeStr=boolean
  ToSeconds : Gain  Gain=sampleTime
  Error : Outport  PortDimensions=1
  wires:
  Logical Operator/1 -> Error/1
  To_ToActuator/1 -> Memory1/1
  Bus Selector/1 -> Logical Operator2/1  "<OperationEnabled>"
  DriveEnable/1 -> Memory/1
  CountHowLongEnableWasTrue/1(y) -> ToSeconds/1
  ToSeconds/1 -> Relational Operator/1
  Relational Operator/1 -> Logical Operator/1
  InhibitTime_s/1 -> Relational Operator/2
  Memory/1 -> CountHowLongEnableWasTrue/1(u)
  Memory1/1 -> Bus Selector/1
  Logical Operator2/1 -> Logical Operator/2

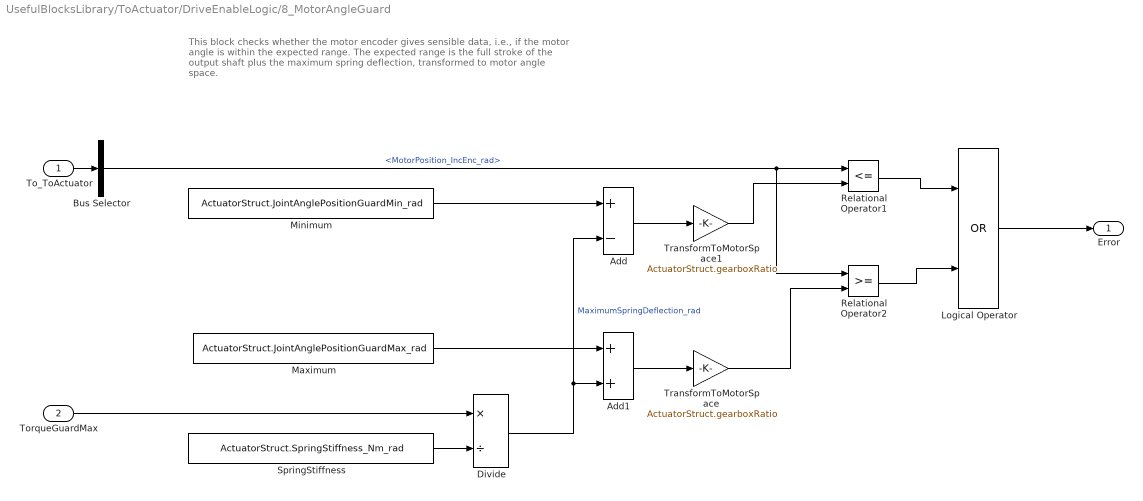
== system UsefulBlocksLibrary/ToActuator/DriveEnableLogic/8_MotorAngleGuard ==
  note: This block checks whether the motor encoder gives sensible data, i.e., if the motor angle is within the expected range. The expected range is the full stroke of the output shaft plus the maximum spring deflection, transformed to motor angle space.
  To_ToActuator : Inport
  TorqueGuardMax : Inport  Port=2
  Add : Sum  Inputs=+-
  Add1 : Sum
  Bus Selector : BusSelector  OutputSignals=MotorPosition_IncEnc_rad
  Divide : Product  Inputs=*/
  Logical Operator : Logic  Operator=OR  AllPortsSameDT=off  OutDataTypeStr=boolean
  Maximum : Constant  Value=ActuatorStruct.JointAnglePositionGuardMax_rad
  Minimum : Constant  Value=ActuatorStruct.JointAnglePositionGuardMin_rad
  Relational Operator1 : RelationalOperator  Operator=<=  OutDataTypeStr=boolean
  Relational Operator2 : RelationalOperator  OutDataTypeStr=boolean
  SpringStiffness : Constant  Value=ActuatorStruct.SpringStiffness_Nm_rad
  TransformToMotorSpace : Gain  Gain=ActuatorStruct.gearboxRatio
  TransformToMotorSpace1 : Gain  Gain=ActuatorStruct.gearboxRatio
  Error : Outport
  wires:
  To_ToActuator/1 -> Bus Selector/1
  Bus Selector/1 -> Relational Operator2/1, Relational Operator1/1  "<MotorPosition_IncEnc_rad>"
  Relational Operator1/1 -> Logical Operator/1
  Relational Operator2/1 -> Logical Operator/2
  Logical Operator/1 -> Error/1
  TransformToMotorSpace1/1 -> Relational Operator1/2
  Add1/1 -> TransformToMotorSpace/1
  Add/1 -> TransformToMotorSpace1/1
  TransformToMotorSpace/1 -> Relational Operator2/2
  TorqueGuardMax/1 -> Divide/1
  SpringStiffness/1 -> Divide/2
  Maximum/1 -> Add1/1
  Divide/1 -> Add/2, Add1/2  "MaximumSpringDeflection_rad"
  Minimum/1 -> Add/1

== system UsefulBlocksLibrary/ToActuator/DriveEnableLogic/CreateSingleErrorValue ==
  ErrorChecks : Inport
  Data Type Conversion1 : DataTypeConversion  OutDataTypeStr=double
  Data Type Conversion2 : DataTypeConversion  OutDataTypeStr=int32
  MATLAB Function : MATLAB Function  TreatAsAtomicUnit=on
  Select_NotUseActuator : Selector  InputPortWidth=3
  Switch : Switch  Criteria=u2 ~= 0
  Unary Minus : UnaryMinus
  Out1 : Outport
  wires:
  Data Type Conversion2/1 -> Switch/3, Unary Minus/1
  MATLAB Function/1(out) -> Data Type Conversion2/1
  Data Type Conversion1/1 -> MATLAB Function/1(errors), Select_NotUseActuator/1
  Select_NotUseActuator/1 -> Switch/2
  ErrorChecks/1 -> Data Type Conversion1/1
  Switch/1 -> Out1/1
  Unary Minus/1 -> Switch/1

== system UsefulBlocksLibrary/ToActuator/DriveEnableLogic/LatchRising ==
  in : Inport
  Trigger : TriggerPort  PortDimensions=1
  out : Outport
  wires:
  in/1 -> out/1

== system UsefulBlocksLibrary/ToActuator/DriveEnableLogic/LatchRising1 ==
  in : Inport
  Trigger : TriggerPort  PortDimensions=1
  out : Outport
  wires:
  in/1 -> out/1

== matlab function UsefulBlocksLibrary/FilterFourthOrder/Filter1 ==
  data: x input; OmegaFilter input; y output; sampleTime parameter
function y = Filter2ndOrder(x, OmegaFilter, sampleTime)
%#codegen

persistent yd_prev y_prev;
if isempty(yd_prev)
    yd_prev = 0; 
    y_prev = 0; %Derivative of the above signal
end;

% Do 2nd order filtering with given omega and zeta=0.7; input of filter
% is vel_inc_sampleTime_unfilt; output is y (we assign to vel_inc_s
% later). 
if OmegaFilter==0 || isinf(OmegaFilter)
    y=x;
    y_prev=y;
    yd_prev =0;
else
    zeta = 0.7;
    ydd = OmegaFilter^2 * (x - y_prev) - 2*zeta*OmegaFilter* yd_prev;
    yd = yd_prev + ydd * sampleTime;
    y = y_prev + yd * sampleTime;

    y_prev = y; yd_prev = yd;
end;

== matlab function UsefulBlocksLibrary/FromActuator/DecodeActualTorque1 ==
  data: JointTorque_Act_Nm output; MotorCurrent_Act_IU input int16; transmissionRatio parameter; drivePeakCurrent parameter; motorTorqueConstant parameter
function JointTorque_Act_Nm = DecodeActualTorque(MotorCurrent_Act_IU, transmissionRatio, drivePeakCurrent, motorTorqueConstant)
%#codegen
%

% convert incremental units to motor torque value. See the technosoft CoE
% manual for the decoding
torquemotor_act = motorTorqueConstant * (double(MotorCurrent_Act_IU)*2*drivePeakCurrent / 65520);

% motor torque to joint torque (transmission). Negate due to sign change
% due to transmission.
JointTorque_Act_Nm = torquemotor_act * transmissionRatio;

== matlab function UsefulBlocksLibrary/ToActuator/DriveEnableLogic/64_DriveError/CountHowLongEnableWasTrue ==
  data: u input; y output
function y = fcn(u)
%#codegen
%
% This block counts how many samples the input has been on (true). As soon
% as the input goes false, the counter is reset.
persistent onCounter;

if isempty(onCounter)
    onCounter = 0;
end;

if u == 1
    onCounter = onCounter + 1;
else
    % u == 0
    onCounter = 0;
end;
y = onCounter;

== matlab function UsefulBlocksLibrary/EncodeDesiredTorque ==
  data: MotorTorque_Des_IU output int16; JointTorque_Des_Nm input; transmissionRatio parameter; motorTorqueConstant parameter; drivePeakCurrent parameter
function MotorTorque_Des_IU = EncodeDesiredTorque(JointTorque_Des_Nm, transmissionRatio, motorTorqueConstant, drivePeakCurrent)
%#codegen
% Calculate the target torque in incremental units for a desired joint
% torque.

% compute torque at motor (negate because sign change due to transmission)
torque_motor = JointTorque_Des_Nm / transmissionRatio; 

% desired current (i_des) = torque_motor / kt (torque constant)
i_des = torque_motor / motorTorqueConstant;

% calculate the target torque in incremental units [IU], see CoE manual
% Technosoftmotion
MotorTorque_Des_IU = int16( 65520*i_des / (2*drivePeakCurrent) );

== matlab function UsefulBlocksLibrary/DecodeActualTorque ==
  data: JointTorque_Act_Nm output; MotorCurrent_Act_IU input int16; transmissionRatio parameter; drivePeakCurrent parameter; motorTorqueConstant parameter
function JointTorque_Act_Nm = DecodeActualTorque(MotorCurrent_Act_IU, transmissionRatio, drivePeakCurrent, motorTorqueConstant)
%#codegen
%

% convert incremental units to motor torque value. See the technosoft CoE
% manual for the decoding
torquemotor_act = motorTorqueConstant * (double(MotorCurrent_Act_IU)*2*drivePeakCurrent / 65520);

% motor torque to joint torque (transmission). Negate due to sign change
% due to transmission.
JointTorque_Act_Nm = torquemotor_act * transmissionRatio;

== matlab function UsefulBlocksLibrary/FilterFourthOrder/Filter2 ==
  data: x input; OmegaFilter input; y output; sampleTime parameter
function y = Filter2ndOrder(x, OmegaFilter, sampleTime)
%#codegen

persistent yd_prev y_prev;
if isempty(yd_prev)
    yd_prev = 0; 
    y_prev = 0; %Derivative of the above signal
end;

% Do 2nd order filtering with given omega and zeta=0.7; input of filter
% is vel_inc_sampleTime_unfilt; output is y (we assign to vel_inc_s
% later). 
if OmegaFilter==0 || isinf(OmegaFilter)
    y=x;
    y_prev=y;
    yd_prev =0;
else
    zeta = 0.7;
    ydd = OmegaFilter^2 * (x - y_prev) - 2*zeta*OmegaFilter* yd_prev;
    yd = yd_prev + ydd * sampleTime;
    y = y_prev + yd * sampleTime;

    y_prev = y; yd_prev = yd;
end;
